simulink subsystem "Plant_v2"  (R2024b)
settings: Solver=VariableStepAuto  StartTime=0.0  StopTime=10.0  RelTol=1e-3
undefined symbols (not defined in the file or in its folder): deadtime_mdot, deadtime_Pc, DiscIntNeverNeededParam, ipa_tank, noise_T, ox_tank, timeDelta, x0
libraries: simulink x5
settings Model: Creator=rober  LastModifiedBy=pplat

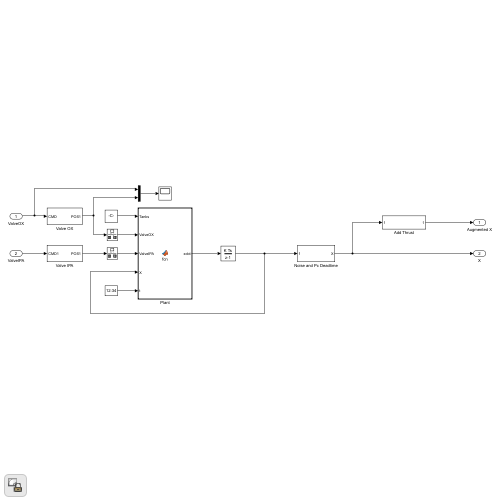
[thumbnail: Simulink's stored preview of the top-level diagram]
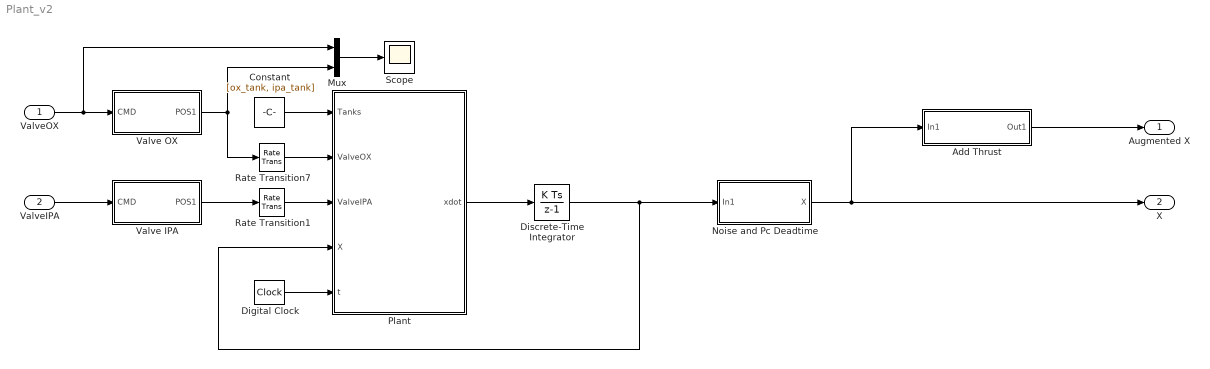
== system Plant_v2 ==
  ValveOX : Inport
  ValveIPA : Inport  Port=2
  Add Thrust : Subsystem
  Constant : Constant  Value=[ox_tank, ipa_tank]
  Digital Clock : DigitalClock  SampleTime=timeDelta
  Discrete-Time Integrator : DiscreteIntegrator  InitialCondition=x0.'  SampleTime=-1  ICPrevOutput=DiscIntNeverNeededParam  ICPrevScaledInput=DiscIntNeverNeededParam
  Mux : Mux  Inputs=2
  Noise and Pc Deadtime : Subsystem
  Plant : MATLAB Function  TreatAsAtomicUnit=on
  Rate Transition1 : RateTransition  OutPortSampleTime=timeDeltaCMD
  Rate Transition7 : RateTransition  OutPortSampleTime=timeDeltaCMD
  Scope : Scope
  Valve IPA : Subsystem
  Valve OX : Subsystem
  Augmented X : Outport
  X : Outport  Port=2
  wires:
  Plant/1(xdot) -> Discrete-Time Integrator/1
  Digital Clock/1 -> Plant/5(t)
  Discrete-Time Integrator/1 -> Noise and Pc Deadtime/1(In1), Plant/4(X)
  Noise and Pc Deadtime/1(X) -> Add Thrust/1(In1), X/1
  Add Thrust/1(Out1) -> Augmented X/1
  Constant/1 -> Plant/1(Tanks)
  ValveOX/1 -> Valve OX/1(CMD), Mux/1
  ValveIPA/1 -> Valve IPA/1(CMD)
  Valve OX/1(POS1) -> Rate Transition7/1, Mux/2
  Valve IPA/1(POS1) -> Rate Transition1/1
  Mux/1 -> Scope/1
  Rate Transition7/1 -> Plant/2(ValveOX)
  Rate Transition1/1 -> Plant/3(ValveIPA)

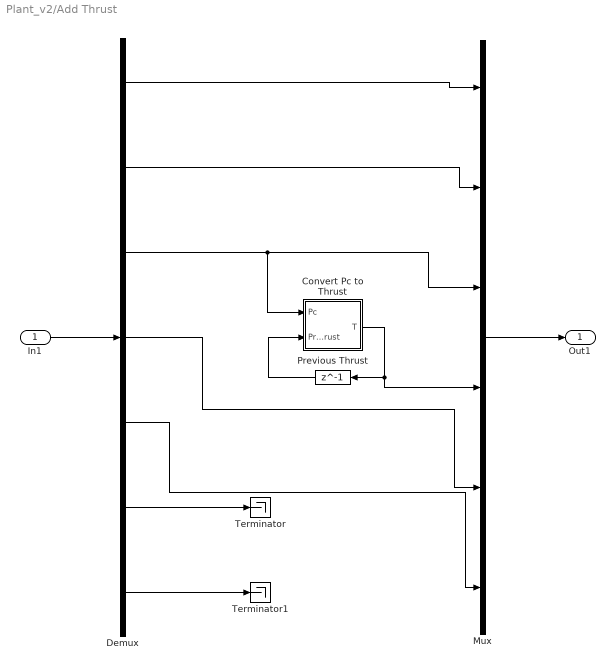
== system Plant_v2/Add Thrust ==
  In1 : Inport
  Convert Pc to Thrust : Subsystem
  Demux : Demux  Outputs=7
  Mux : Mux  Inputs=6
  Previous Thrust : Delay  DelayLength=1
  Terminator : Terminator
  Terminator1 : Terminator
  Out1 : Outport
  wires:
  Demux/7 -> Terminator1/1
  Demux/6 -> Terminator/1
  Demux/4 -> Mux/5
  Demux/5 -> Mux/6
  Convert Pc to Thrust/1(T) -> Previous Thrust/1, Mux/4
  Previous Thrust/1 -> Convert Pc to Thrust/2(PrevThrust)
  Demux/3 -> Mux/3, Convert Pc to Thrust/1(Pc)
  In1/1 -> Demux/1
  Mux/1 -> Out1/1
  Demux/2 -> Mux/2
  Demux/1 -> Mux/1

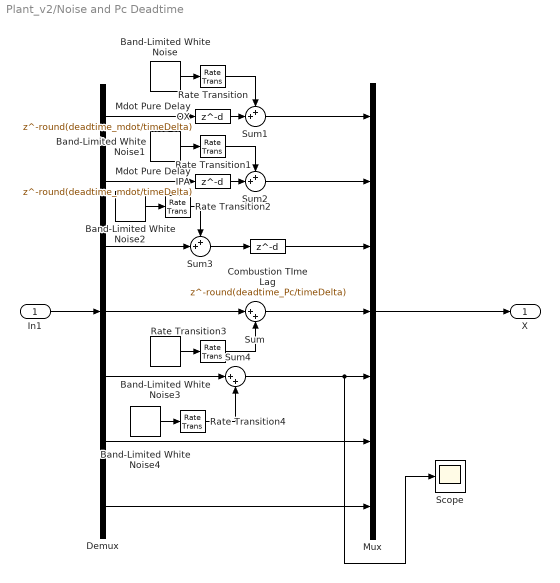
== system Plant_v2/Noise and Pc Deadtime ==
  In1 : Inport  SampleTime=timeDelta
  Band-Limited White Noise : simulink/Sources/Band-Limited White Noise  Cov=noise_var_mdot  Ts=noise_T  seed=[23341]
      link override White Noise: SampleTime=0.0002
  Band-Limited White Noise1 : simulink/Sources/Band-Limited White Noise  Cov=noise_var_mdot  Ts=noise_T  seed=[23341]
      link override White Noise: SampleTime=0.0002
  Band-Limited White Noise2 : simulink/Sources/Band-Limited White Noise  Cov=noise_var_pc  Ts=noise_T  seed=[23341]
      link override White Noise: SampleTime=0.0002
  Band-Limited White Noise3 : simulink/Sources/Band-Limited White Noise  Cov=noise_var_pout  Ts=noise_T  seed=[23341]
      link override White Noise: SampleTime=-1
  Band-Limited White Noise4 : simulink/Sources/Band-Limited White Noise  Cov=noise_var_pout  Ts=noise_T  seed=[23341]
      link override White Noise: SampleTime=-1
  Combustion TIme Lag : Delay  DelayLength=round(deadtime_Pc/timeDelta)  InitialCondition=x0(3)
  Demux : Demux  Outputs=7
  Mdot Pure Delay IPA : Delay  DelayLength=round(deadtime_mdot/timeDelta)  SampleTime=timeDelta
  Mdot Pure Delay OX : Delay  DelayLength=round(deadtime_mdot/timeDelta)  SampleTime=timeDelta
  Mux : Mux  Inputs=7
  Rate Transition{,1..4} (5 alike) : RateTransition  OutPortSampleTime=timeDelta
  Scope : Scope
  Sum : Sum  Inputs=|++
  Sum1 : Sum  Inputs=++|
  Sum2 : Sum  Inputs=++|
  Sum3 : Sum  Inputs=++|
  Sum4 : Sum  Inputs=|++
  X : Outport  PortDimensions=7
  wires:
  Demux/7 -> Mux/7
  Demux/6 -> Mux/6
  Sum4/1 -> Mux/5, Scope/1
  Sum/1 -> Mux/4
  Demux/1 -> Mdot Pure Delay OX/1
  Sum1/1 -> Mux/1
  Demux/2 -> Mdot Pure Delay IPA/1
  Sum2/1 -> Mux/2
  Combustion TIme Lag/1 -> Mux/3
  Demux/3 -> Sum3/2
  Sum3/1 -> Combustion TIme Lag/1
  Rate Transition4/1 -> Sum4/2
  Rate Transition3/1 -> Sum/2
  Rate Transition2/1 -> Sum3/1
  Rate Transition1/1 -> Sum2/1
  Rate Transition/1 -> Sum1/1
  Mdot Pure Delay OX/1 -> Sum1/2
  Mdot Pure Delay IPA/1 -> Sum2/2
  Band-Limited White Noise2/1 -> Rate Transition2/1
  Band-Limited White Noise1/1 -> Rate Transition1/1
  Band-Limited White Noise/1 -> Rate Transition/1
  In1/1 -> Demux/1
  Mux/1 -> X/1
  Demux/4 -> Sum/1
  Demux/5 -> Sum4/1
  Band-Limited White Noise3/1 -> Rate Transition3/1
  Band-Limited White Noise4/1 -> Rate Transition4/1

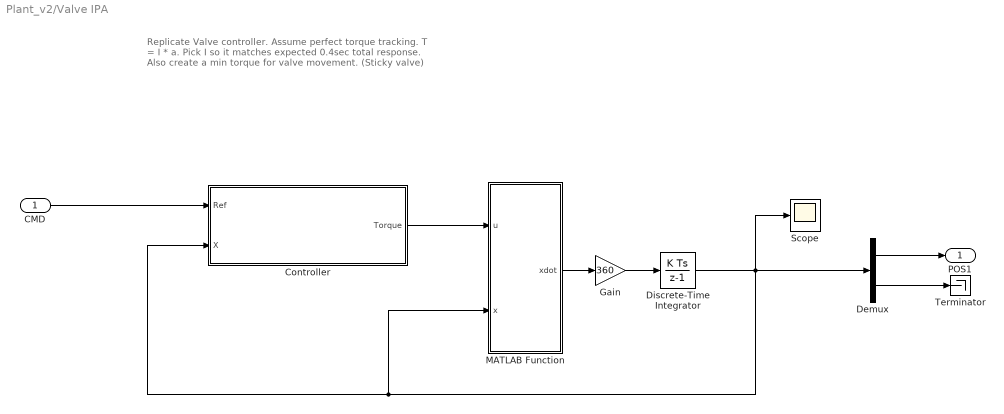
== system Plant_v2/Valve IPA ==
  note: Replicate Valve controller. Assume perfect
      | torque tracking.  T = I * a. Pick I so it matches
      | expected 0.4sec total response. Also create a
      | min torque for valve movement. (Sticky valve)
  CMD : Inport
  Controller : Subsystem
  Demux : Demux  Outputs=2
  Discrete-Time Integrator : DiscreteIntegrator  InitialCondition=[x0(7), 0]  SampleTime=-1  ICPrevOutput=DiscIntNeverNeededParam  ICPrevScaledInput=DiscIntNeverNeededParam
  Gain : Gain  Gain=360
  MATLAB Function : MATLAB Function  TreatAsAtomicUnit=on
  Scope : Scope
  Terminator : Terminator
  POS1 : Outport
  wires:
  Gain/1 -> Discrete-Time Integrator/1
  Discrete-Time Integrator/1 -> MATLAB Function/2(x), Controller/2(X), Demux/1, Scope/1
  Demux/2 -> Terminator/1
  Demux/1 -> POS1/1
  Controller/1(Torque) -> MATLAB Function/1(u)
  CMD/1 -> Controller/1(Ref)
  MATLAB Function/1(xdot) -> Gain/1

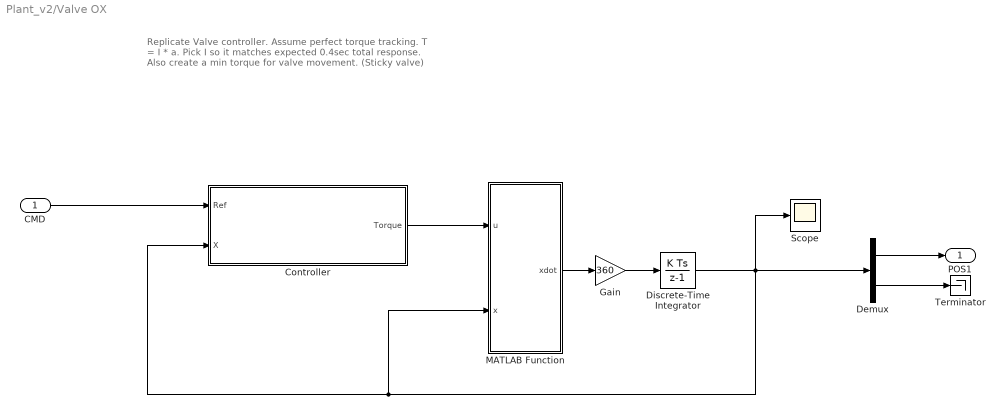
== system Plant_v2/Valve OX ==
  note: Replicate Valve controller. Assume perfect
      | torque tracking.  T = I * a. Pick I so it matches
      | expected 0.4sec total response. Also create a
      | min torque for valve movement. (Sticky valve)
  CMD : Inport
  Controller : Subsystem
  Demux : Demux  Outputs=2
  Discrete-Time Integrator : DiscreteIntegrator  InitialCondition=[x0(6), 0]  SampleTime=-1  ICPrevOutput=DiscIntNeverNeededParam  ICPrevScaledInput=DiscIntNeverNeededParam
  Gain : Gain  Gain=360
  MATLAB Function : MATLAB Function  TreatAsAtomicUnit=on
  Scope : Scope
  Terminator : Terminator
  POS1 : Outport
  wires:
  Gain/1 -> Discrete-Time Integrator/1
  Discrete-Time Integrator/1 -> MATLAB Function/2(x), Controller/2(X), Demux/1, Scope/1
  Demux/2 -> Terminator/1
  Demux/1 -> POS1/1
  Controller/1(Torque) -> MATLAB Function/1(u)
  CMD/1 -> Controller/1(Ref)
  MATLAB Function/1(xdot) -> Gain/1

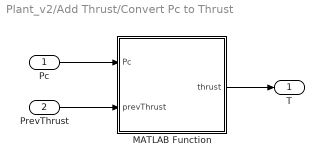
== system Plant_v2/Add Thrust/Convert Pc to Thrust ==
  Pc : Inport
  PrevThrust : Inport  Port=2
  MATLAB Function : MATLAB Function  TreatAsAtomicUnit=on
  T : Outport
  wires:
  MATLAB Function/1(thrust) -> T/1
  Pc/1 -> MATLAB Function/1(Pc)
  PrevThrust/1 -> MATLAB Function/2(prevThrust)

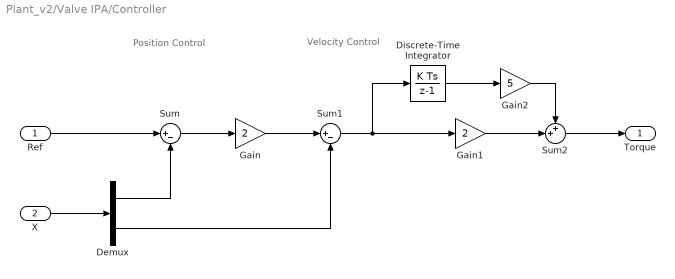
== system Plant_v2/Valve IPA/Controller ==
  note: Velocity Control
  note: Position Control
  Ref : Inport
  X : Inport  Port=2
  Demux : Demux  Outputs=2
  Discrete-Time Integrator : DiscreteIntegrator  SampleTime=-1  ICPrevOutput=DiscIntNeverNeededParam  ICPrevScaledInput=DiscIntNeverNeededParam
  Gain : Gain  Gain=2
  Gain1 : Gain  Gain=2
  Gain2 : Gain  Gain=5
  Sum : Sum  Inputs=|+-
  Sum1 : Sum  Inputs=|+-
  Sum2 : Sum  Inputs=++|
  Torque : Outport
  wires:
  Ref/1 -> Sum/1
  Gain2/1 -> Sum2/1
  Discrete-Time Integrator/1 -> Gain2/1
  Sum2/1 -> Torque/1
  Gain1/1 -> Sum2/2
  Demux/2 -> Sum1/2
  Gain/1 -> Sum1/1
  Sum1/1 -> Gain1/1, Discrete-Time Integrator/1
  Demux/1 -> Sum/2
  Sum/1 -> Gain/1
  X/1 -> Demux/1

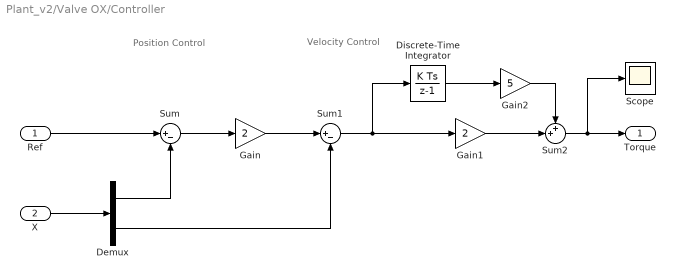
== system Plant_v2/Valve OX/Controller ==
  note: Velocity Control
  note: Position Control
  Ref : Inport
  X : Inport  Port=2
  Demux : Demux  Outputs=2
  Discrete-Time Integrator : DiscreteIntegrator  SampleTime=-1  ICPrevOutput=DiscIntNeverNeededParam  ICPrevScaledInput=DiscIntNeverNeededParam
  Gain : Gain  Gain=2
  Gain1 : Gain  Gain=2
  Gain2 : Gain  Gain=5
  Scope : Scope
  Sum : Sum  Inputs=|+-
  Sum1 : Sum  Inputs=|+-
  Sum2 : Sum  Inputs=++|
  Torque : Outport
  wires:
  Ref/1 -> Sum/1
  Gain2/1 -> Sum2/1
  Discrete-Time Integrator/1 -> Gain2/1
  Sum2/1 -> Torque/1, Scope/1
  Gain1/1 -> Sum2/2
  Demux/2 -> Sum1/2
  Gain/1 -> Sum1/1
  Sum1/1 -> Gain1/1, Discrete-Time Integrator/1
  Demux/1 -> Sum/2
  Sum/1 -> Gain/1
  X/1 -> Demux/1

== matlab function Plant_v2/Add Thrust/Convert Pc to Thrust/MATLAB Function ==
  data: Pc input; prevThrust input; thrust output
function thrust = convertThrust(Pc, prevThrust)

    thrust = cp_to_thrust(Pc, prevThrust);
end

== matlab function Plant_v2/Plant ==
  data: Tanks input; ValveOX input; ValveIPA input; X input; xdot output; t input
function xdot = fcn(Tanks, ValveOX, ValveIPA, X, t)
   
    ox_tank = Tanks(1);
    ipa_tank = Tanks(2);
    xdot = nonlinear_plant3(X, ValveOX, ValveIPA, t, 1, ox_tank, ipa_tank);
end

== matlab function Plant_v2/Valve IPA/MATLAB Function ==
  data: u input; x input; xdot output
function xdot = valve(u, x)

    xdot = valvedynamics(x, u);
end

== matlab function Plant_v2/Valve OX/MATLAB Function ==
  data: u input; x input; xdot output
function xdot = valve(u, x)

    xdot = valvedynamics(x, u);
end
